simulink library "packLibrary"  (R2022b)
settings: Solver=VariableStepAuto  StartTime=0.0  StopTime=10.0  RelTol=1e-3
undefined symbols (not defined in the file or in its folder): battery_builder_rtmsupport, gcbh
libraries: packLibrary_lib x42
(part 4 of 4)

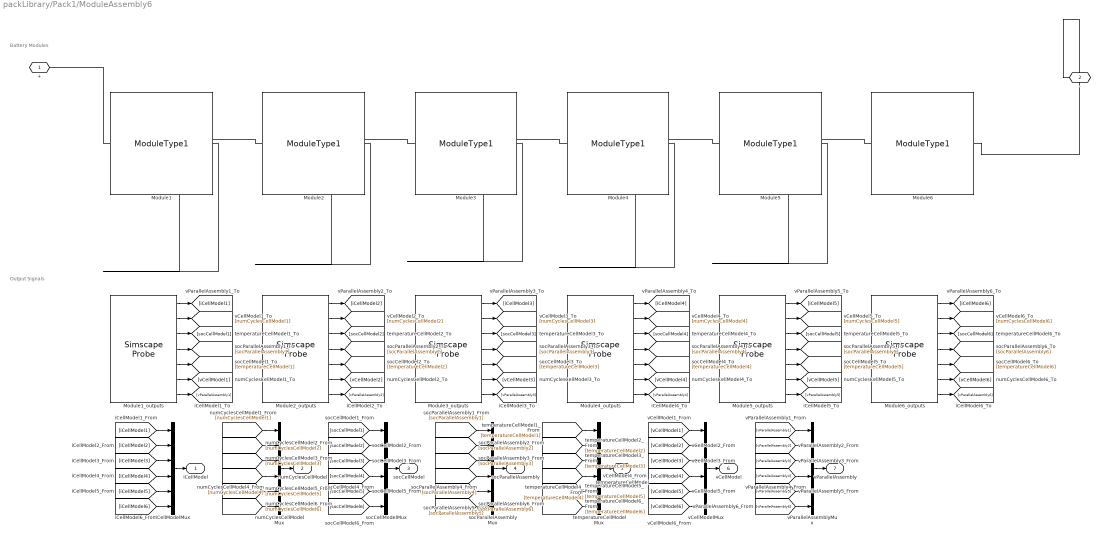
== system packLibrary/Pack1/ModuleAssembly6 ==
  note: Output Signals
  note: Battery Modules
  Module1 : packLibrary_lib/Modules/ModuleType1  SOC_vec=ModuleType1.SOC_vec  T_vec=ModuleType1.T_vec K  V0_mat=ModuleType1.V0_mat V  V_range=ModuleType1.V_range V  R0_mat=ModuleType1.R0_mat Ohm  AH=ModuleType1.AH A*hr  extrapolation_option=simscape.enum.extrapolation.nearest  thermal_mass=ModuleType1.thermal_mass J/K  P=4  S=3  iCellModel_specify=on  iCellModel_priority=None  iCellModel=ModuleAssembly6.Module1.iCellModel A  iCellModel_nominal_specify=off  iCellModel_nominal_unit=A  iCellModel_nominal_value=1  vCellModel_specify=on  vCellModel_priority=None  vCellModel=ModuleAssembly6.Module1.vCellModel V  vCellModel_nominal_specify=off  vCellModel_nominal_unit=V  vCellModel_nominal_value=1  socCellModel_specify=on  socCellModel_priority=High  socCellModel=ModuleAssembly6.Module1.socCellModel  socCellModel_nominal_specify=off  socCellModel_nominal_unit=1  socCellModel_nominal_value=1  numCyclesCellModel_specify=on  numCyclesCellModel_priority=High  numCyclesCellModel=ModuleAssembly6.Module1.numCyclesCellModel  numCyclesCellModel_nominal_specify=off  numCyclesCellModel_nominal_unit=1  numCyclesCellModel_nominal_value=1  temperatureCellModel_specify=on  temperatureCellModel_priority=High  temperatureCellModel=ModuleAssembly6.Module1.temperatureCellModel K  temperatureCellModel_nominal_specify=off  temperatureCellModel_nominal_unit=K  temperatureCellModel_nominal_value=1  vParallelAssembly_specify=on  vParallelAssembly_priority=None  vParallelAssembly=ModuleAssembly6.Module1.vParallelAssembly V  vParallelAssembly_nominal_specify=off  vParallelAssembly_nominal_unit=V  vParallelAssembly_nominal_value=1  socParallelAssembly_specify=on  socParallelAssembly_priority=None  socParallelAssembly=ModuleAssembly6.Module1.socParallelAssembly  socParallelAssembly_nominal_specify=off  socParallelAssembly_nominal_unit=1  socParallelAssembly_nominal_value=1
      settings: InternalSimscapePortConfiguration="{\"Bottom\":[{\"id\":\"n\",\"label\":\"-\",\"type\":\"foundation.electrical.electrical\"}],\"Left\":[],\"Right\":[],\"Top\":[{\"id\":\"p\",\"label\":\"+\",\"type\":\"foundation.electrical.electrical\"}]}"
  Module1_outputs : SimscapeProbe  BoundBlock=694  Variables={iCellModel, numCyclesCellModel, socCellModel, socParallelAssembly, temperatureCellModel, vCellModel, vParallelAssembly}
  Module2 : packLibrary_lib/Modules/ModuleType1  SOC_vec=ModuleType1.SOC_vec  T_vec=ModuleType1.T_vec K  V0_mat=ModuleType1.V0_mat V  V_range=ModuleType1.V_range V  R0_mat=ModuleType1.R0_mat Ohm  AH=ModuleType1.AH A*hr  extrapolation_option=simscape.enum.extrapolation.nearest  thermal_mass=ModuleType1.thermal_mass J/K  P=4  S=3  iCellModel_specify=on  iCellModel_priority=None  iCellModel=ModuleAssembly6.Module2.iCellModel A  iCellModel_nominal_specify=off  iCellModel_nominal_unit=A  iCellModel_nominal_value=1  vCellModel_specify=on  vCellModel_priority=None  vCellModel=ModuleAssembly6.Module2.vCellModel V  vCellModel_nominal_specify=off  vCellModel_nominal_unit=V  vCellModel_nominal_value=1  socCellModel_specify=on  socCellModel_priority=High  socCellModel=ModuleAssembly6.Module2.socCellModel  socCellModel_nominal_specify=off  socCellModel_nominal_unit=1  socCellModel_nominal_value=1  numCyclesCellModel_specify=on  numCyclesCellModel_priority=High  numCyclesCellModel=ModuleAssembly6.Module2.numCyclesCellModel  numCyclesCellModel_nominal_specify=off  numCyclesCellModel_nominal_unit=1  numCyclesCellModel_nominal_value=1  temperatureCellModel_specify=on  temperatureCellModel_priority=High  temperatureCellModel=ModuleAssembly6.Module2.temperatureCellModel K  temperatureCellModel_nominal_specify=off  temperatureCellModel_nominal_unit=K  temperatureCellModel_nominal_value=1  vParallelAssembly_specify=on  vParallelAssembly_priority=None  vParallelAssembly=ModuleAssembly6.Module2.vParallelAssembly V  vParallelAssembly_nominal_specify=off  vParallelAssembly_nominal_unit=V  vParallelAssembly_nominal_value=1  socParallelAssembly_specify=on  socParallelAssembly_priority=None  socParallelAssembly=ModuleAssembly6.Module2.socParallelAssembly  socParallelAssembly_nominal_specify=off  socParallelAssembly_nominal_unit=1  socParallelAssembly_nominal_value=1
      settings: InternalSimscapePortConfiguration="{\"Bottom\":[{\"id\":\"n\",\"label\":\"-\",\"type\":\"foundation.electrical.electrical\"}],\"Left\":[],\"Right\":[],\"Top\":[{\"id\":\"p\",\"label\":\"+\",\"type\":\"foundation.electrical.electrical\"}]}"
  Module2_outputs : SimscapeProbe  BoundBlock=696  Variables={iCellModel, numCyclesCellModel, socCellModel, socParallelAssembly, temperatureCellModel, vCellModel, vParallelAssembly}
  Module3 : packLibrary_lib/Modules/ModuleType1  SOC_vec=ModuleType1.SOC_vec  T_vec=ModuleType1.T_vec K  V0_mat=ModuleType1.V0_mat V  V_range=ModuleType1.V_range V  R0_mat=ModuleType1.R0_mat Ohm  AH=ModuleType1.AH A*hr  extrapolation_option=simscape.enum.extrapolation.nearest  thermal_mass=ModuleType1.thermal_mass J/K  P=4  S=3  iCellModel_specify=on  iCellModel_priority=None  iCellModel=ModuleAssembly6.Module3.iCellModel A  iCellModel_nominal_specify=off  iCellModel_nominal_unit=A  iCellModel_nominal_value=1  vCellModel_specify=on  vCellModel_priority=None  vCellModel=ModuleAssembly6.Module3.vCellModel V  vCellModel_nominal_specify=off  vCellModel_nominal_unit=V  vCellModel_nominal_value=1  socCellModel_specify=on  socCellModel_priority=High  socCellModel=ModuleAssembly6.Module3.socCellModel  socCellModel_nominal_specify=off  socCellModel_nominal_unit=1  socCellModel_nominal_value=1  numCyclesCellModel_specify=on  numCyclesCellModel_priority=High  numCyclesCellModel=ModuleAssembly6.Module3.numCyclesCellModel  numCyclesCellModel_nominal_specify=off  numCyclesCellModel_nominal_unit=1  numCyclesCellModel_nominal_value=1  temperatureCellModel_specify=on  temperatureCellModel_priority=High  temperatureCellModel=ModuleAssembly6.Module3.temperatureCellModel K  temperatureCellModel_nominal_specify=off  temperatureCellModel_nominal_unit=K  temperatureCellModel_nominal_value=1  vParallelAssembly_specify=on  vParallelAssembly_priority=None  vParallelAssembly=ModuleAssembly6.Module3.vParallelAssembly V  vParallelAssembly_nominal_specify=off  vParallelAssembly_nominal_unit=V  vParallelAssembly_nominal_value=1  socParallelAssembly_specify=on  socParallelAssembly_priority=None  socParallelAssembly=ModuleAssembly6.Module3.socParallelAssembly  socParallelAssembly_nominal_specify=off  socParallelAssembly_nominal_unit=1  socParallelAssembly_nominal_value=1
      settings: InternalSimscapePortConfiguration="{\"Bottom\":[{\"id\":\"n\",\"label\":\"-\",\"type\":\"foundation.electrical.electrical\"}],\"Left\":[],\"Right\":[],\"Top\":[{\"id\":\"p\",\"label\":\"+\",\"type\":\"foundation.electrical.electrical\"}]}"
  Module3_outputs : SimscapeProbe  BoundBlock=698  Variables={iCellModel, numCyclesCellModel, socCellModel, socParallelAssembly, temperatureCellModel, vCellModel, vParallelAssembly}
  Module4 : packLibrary_lib/Modules/ModuleType1  SOC_vec=ModuleType1.SOC_vec  T_vec=ModuleType1.T_vec K  V0_mat=ModuleType1.V0_mat V  V_range=ModuleType1.V_range V  R0_mat=ModuleType1.R0_mat Ohm  AH=ModuleType1.AH A*hr  extrapolation_option=simscape.enum.extrapolation.nearest  thermal_mass=ModuleType1.thermal_mass J/K  P=4  S=3  iCellModel_specify=on  iCellModel_priority=None  iCellModel=ModuleAssembly6.Module4.iCellModel A  iCellModel_nominal_specify=off  iCellModel_nominal_unit=A  iCellModel_nominal_value=1  vCellModel_specify=on  vCellModel_priority=None  vCellModel=ModuleAssembly6.Module4.vCellModel V  vCellModel_nominal_specify=off  vCellModel_nominal_unit=V  vCellModel_nominal_value=1  socCellModel_specify=on  socCellModel_priority=High  socCellModel=ModuleAssembly6.Module4.socCellModel  socCellModel_nominal_specify=off  socCellModel_nominal_unit=1  socCellModel_nominal_value=1  numCyclesCellModel_specify=on  numCyclesCellModel_priority=High  numCyclesCellModel=ModuleAssembly6.Module4.numCyclesCellModel  numCyclesCellModel_nominal_specify=off  numCyclesCellModel_nominal_unit=1  numCyclesCellModel_nominal_value=1  temperatureCellModel_specify=on  temperatureCellModel_priority=High  temperatureCellModel=ModuleAssembly6.Module4.temperatureCellModel K  temperatureCellModel_nominal_specify=off  temperatureCellModel_nominal_unit=K  temperatureCellModel_nominal_value=1  vParallelAssembly_specify=on  vParallelAssembly_priority=None  vParallelAssembly=ModuleAssembly6.Module4.vParallelAssembly V  vParallelAssembly_nominal_specify=off  vParallelAssembly_nominal_unit=V  vParallelAssembly_nominal_value=1  socParallelAssembly_specify=on  socParallelAssembly_priority=None  socParallelAssembly=ModuleAssembly6.Module4.socParallelAssembly  socParallelAssembly_nominal_specify=off  socParallelAssembly_nominal_unit=1  socParallelAssembly_nominal_value=1
      settings: InternalSimscapePortConfiguration="{\"Bottom\":[{\"id\":\"n\",\"label\":\"-\",\"type\":\"foundation.electrical.electrical\"}],\"Left\":[],\"Right\":[],\"Top\":[{\"id\":\"p\",\"label\":\"+\",\"type\":\"foundation.electrical.electrical\"}]}"
  Module4_outputs : SimscapeProbe  BoundBlock=700  Variables={iCellModel, numCyclesCellModel, socCellModel, socParallelAssembly, temperatureCellModel, vCellModel, vParallelAssembly}
  Module5 : packLibrary_lib/Modules/ModuleType1  SOC_vec=ModuleType1.SOC_vec  T_vec=ModuleType1.T_vec K  V0_mat=ModuleType1.V0_mat V  V_range=ModuleType1.V_range V  R0_mat=ModuleType1.R0_mat Ohm  AH=ModuleType1.AH A*hr  extrapolation_option=simscape.enum.extrapolation.nearest  thermal_mass=ModuleType1.thermal_mass J/K  P=4  S=3  iCellModel_specify=on  iCellModel_priority=None  iCellModel=ModuleAssembly6.Module5.iCellModel A  iCellModel_nominal_specify=off  iCellModel_nominal_unit=A  iCellModel_nominal_value=1  vCellModel_specify=on  vCellModel_priority=None  vCellModel=ModuleAssembly6.Module5.vCellModel V  vCellModel_nominal_specify=off  vCellModel_nominal_unit=V  vCellModel_nominal_value=1  socCellModel_specify=on  socCellModel_priority=High  socCellModel=ModuleAssembly6.Module5.socCellModel  socCellModel_nominal_specify=off  socCellModel_nominal_unit=1  socCellModel_nominal_value=1  numCyclesCellModel_specify=on  numCyclesCellModel_priority=High  numCyclesCellModel=ModuleAssembly6.Module5.numCyclesCellModel  numCyclesCellModel_nominal_specify=off  numCyclesCellModel_nominal_unit=1  numCyclesCellModel_nominal_value=1  temperatureCellModel_specify=on  temperatureCellModel_priority=High  temperatureCellModel=ModuleAssembly6.Module5.temperatureCellModel K  temperatureCellModel_nominal_specify=off  temperatureCellModel_nominal_unit=K  temperatureCellModel_nominal_value=1  vParallelAssembly_specify=on  vParallelAssembly_priority=None  vParallelAssembly=ModuleAssembly6.Module5.vParallelAssembly V  vParallelAssembly_nominal_specify=off  vParallelAssembly_nominal_unit=V  vParallelAssembly_nominal_value=1  socParallelAssembly_specify=on  socParallelAssembly_priority=None  socParallelAssembly=ModuleAssembly6.Module5.socParallelAssembly  socParallelAssembly_nominal_specify=off  socParallelAssembly_nominal_unit=1  socParallelAssembly_nominal_value=1
      settings: InternalSimscapePortConfiguration="{\"Bottom\":[{\"id\":\"n\",\"label\":\"-\",\"type\":\"foundation.electrical.electrical\"}],\"Left\":[],\"Right\":[],\"Top\":[{\"id\":\"p\",\"label\":\"+\",\"type\":\"foundation.electrical.electrical\"}]}"
  Module5_outputs : SimscapeProbe  BoundBlock=702  Variables={iCellModel, numCyclesCellModel, socCellModel, socParallelAssembly, temperatureCellModel, vCellModel, vParallelAssembly}
  Module6 : packLibrary_lib/Modules/ModuleType1  SOC_vec=ModuleType1.SOC_vec  T_vec=ModuleType1.T_vec K  V0_mat=ModuleType1.V0_mat V  V_range=ModuleType1.V_range V  R0_mat=ModuleType1.R0_mat Ohm  AH=ModuleType1.AH A*hr  extrapolation_option=simscape.enum.extrapolation.nearest  thermal_mass=ModuleType1.thermal_mass J/K  P=4  S=3  iCellModel_specify=on  iCellModel_priority=None  iCellModel=ModuleAssembly6.Module6.iCellModel A  iCellModel_nominal_specify=off  iCellModel_nominal_unit=A  iCellModel_nominal_value=1  vCellModel_specify=on  vCellModel_priority=None  vCellModel=ModuleAssembly6.Module6.vCellModel V  vCellModel_nominal_specify=off  vCellModel_nominal_unit=V  vCellModel_nominal_value=1  socCellModel_specify=on  socCellModel_priority=High  socCellModel=ModuleAssembly6.Module6.socCellModel  socCellModel_nominal_specify=off  socCellModel_nominal_unit=1  socCellModel_nominal_value=1  numCyclesCellModel_specify=on  numCyclesCellModel_priority=High  numCyclesCellModel=ModuleAssembly6.Module6.numCyclesCellModel  numCyclesCellModel_nominal_specify=off  numCyclesCellModel_nominal_unit=1  numCyclesCellModel_nominal_value=1  temperatureCellModel_specify=on  temperatureCellModel_priority=High  temperatureCellModel=ModuleAssembly6.Module6.temperatureCellModel K  temperatureCellModel_nominal_specify=off  temperatureCellModel_nominal_unit=K  temperatureCellModel_nominal_value=1  vParallelAssembly_specify=on  vParallelAssembly_priority=None  vParallelAssembly=ModuleAssembly6.Module6.vParallelAssembly V  vParallelAssembly_nominal_specify=off  vParallelAssembly_nominal_unit=V  vParallelAssembly_nominal_value=1  socParallelAssembly_specify=on  socParallelAssembly_priority=None  socParallelAssembly=ModuleAssembly6.Module6.socParallelAssembly  socParallelAssembly_nominal_specify=off  socParallelAssembly_nominal_unit=1  socParallelAssembly_nominal_value=1
      settings: InternalSimscapePortConfiguration="{\"Bottom\":[{\"id\":\"n\",\"label\":\"-\",\"type\":\"foundation.electrical.electrical\"}],\"Left\":[],\"Right\":[],\"Top\":[{\"id\":\"p\",\"label\":\"+\",\"type\":\"foundation.electrical.electrical\"}]}"
  Module6_outputs : SimscapeProbe  BoundBlock=704  Variables={iCellModel, numCyclesCellModel, socCellModel, socParallelAssembly, temperatureCellModel, vCellModel, vParallelAssembly}
  iCellModelMux : Mux  Inputs=6
  numCyclesCellModelMux : Mux  Inputs=6
  socCellModelMux : Mux  Inputs=6
  socParallelAssemblyMux : Mux  Inputs=6
  temperatureCellModelMux : Mux  Inputs=6
  vCellModelMux : Mux  Inputs=6
  vParallelAssemblyMux : Mux  Inputs=6
  + : PMIOPort  Side=Left
  - : PMIOPort  Port=2  Side=Right
  iCellModel : Outport
  numCyclesCellModel : Outport  Port=2
  socCellModel : Outport  Port=3
  socParallelAssembly : Outport  Port=4
  temperatureCellModel : Outport  Port=5
  vCellModel : Outport  Port=6
  vParallelAssembly : Outport  Port=7
  wires:
  [vParallelAssembly6] -> vParallelAssemblyMux/6
  Module6_outputs/1 -> [iCellModel6]
  [vCellModel6] -> vCellModelMux/6
  Module6_outputs/2 -> [numCyclesCellModel6]
  [temperatureCellModel6] -> temperatureCellModelMux/6
  Module6_outputs/3 -> [socCellModel6]
  [socParallelAssembly6] -> socParallelAssemblyMux/6
  Module6_outputs/4 -> [socParallelAssembly6]
  [socCellModel6] -> socCellModelMux/6
  Module6_outputs/5 -> [temperatureCellModel6]
  [numCyclesCellModel6] -> numCyclesCellModelMux/6
  Module6_outputs/6 -> [vCellModel6]
  [iCellModel6] -> iCellModelMux/6
  Module6_outputs/7 -> [vParallelAssembly6]
  [vParallelAssembly5] -> vParallelAssemblyMux/5
  Module5_outputs/1 -> [iCellModel5]
  [vCellModel5] -> vCellModelMux/5
  Module5_outputs/2 -> [numCyclesCellModel5]
  [temperatureCellModel5] -> temperatureCellModelMux/5
  Module5_outputs/3 -> [socCellModel5]
  [socParallelAssembly5] -> socParallelAssemblyMux/5
  Module5_outputs/4 -> [socParallelAssembly5]
  [socCellModel5] -> socCellModelMux/5
  Module5_outputs/5 -> [temperatureCellModel5]
  [numCyclesCellModel5] -> numCyclesCellModelMux/5
  Module5_outputs/6 -> [vCellModel5]
  [iCellModel5] -> iCellModelMux/5
  Module5_outputs/7 -> [vParallelAssembly5]
  [vParallelAssembly4] -> vParallelAssemblyMux/4
  Module4_outputs/1 -> [iCellModel4]
  [vCellModel4] -> vCellModelMux/4
  Module4_outputs/2 -> [numCyclesCellModel4]
  [temperatureCellModel4] -> temperatureCellModelMux/4
  Module4_outputs/3 -> [socCellModel4]
  [socParallelAssembly4] -> socParallelAssemblyMux/4
  Module4_outputs/4 -> [socParallelAssembly4]
  [socCellModel4] -> socCellModelMux/4
  Module4_outputs/5 -> [temperatureCellModel4]
  [numCyclesCellModel4] -> numCyclesCellModelMux/4
  Module4_outputs/6 -> [vCellModel4]
  [iCellModel4] -> iCellModelMux/4
  Module4_outputs/7 -> [vParallelAssembly4]
  [vParallelAssembly3] -> vParallelAssemblyMux/3
  Module3_outputs/1 -> [iCellModel3]
  [vCellModel3] -> vCellModelMux/3
  Module3_outputs/2 -> [numCyclesCellModel3]
  [temperatureCellModel3] -> temperatureCellModelMux/3
  Module3_outputs/3 -> [socCellModel3]
  [socParallelAssembly3] -> socParallelAssemblyMux/3
  Module3_outputs/4 -> [socParallelAssembly3]
  [socCellModel3] -> socCellModelMux/3
  Module3_outputs/5 -> [temperatureCellModel3]
  [numCyclesCellModel3] -> numCyclesCellModelMux/3
  Module3_outputs/6 -> [vCellModel3]
  [iCellModel3] -> iCellModelMux/3
  Module3_outputs/7 -> [vParallelAssembly3]
  [vParallelAssembly2] -> vParallelAssemblyMux/2
  Module2_outputs/1 -> [iCellModel2]
  [vCellModel2] -> vCellModelMux/2
  Module2_outputs/2 -> [numCyclesCellModel2]
  [temperatureCellModel2] -> temperatureCellModelMux/2
  Module2_outputs/3 -> [socCellModel2]
  [socParallelAssembly2] -> socParallelAssemblyMux/2
  Module2_outputs/4 -> [socParallelAssembly2]
  [socCellModel2] -> socCellModelMux/2
  Module2_outputs/5 -> [temperatureCellModel2]
  [numCyclesCellModel2] -> numCyclesCellModelMux/2
  Module2_outputs/6 -> [vCellModel2]
  [iCellModel2] -> iCellModelMux/2
  Module2_outputs/7 -> [vParallelAssembly2]
  [vParallelAssembly1] -> vParallelAssemblyMux/1
  vParallelAssemblyMux/1 -> vParallelAssembly/1
  Module1_outputs/1 -> [iCellModel1]
  [vCellModel1] -> vCellModelMux/1
  vCellModelMux/1 -> vCellModel/1
  Module1_outputs/2 -> [numCyclesCellModel1]
  [temperatureCellModel1] -> temperatureCellModelMux/1
  temperatureCellModelMux/1 -> temperatureCellModel/1
  Module1_outputs/3 -> [socCellModel1]
  [socParallelAssembly1] -> socParallelAssemblyMux/1
  socParallelAssemblyMux/1 -> socParallelAssembly/1
  Module1_outputs/4 -> [socParallelAssembly1]
  [socCellModel1] -> socCellModelMux/1
  socCellModelMux/1 -> socCellModel/1
  Module1_outputs/5 -> [temperatureCellModel1]
  [numCyclesCellModel1] -> numCyclesCellModelMux/1
  numCyclesCellModelMux/1 -> numCyclesCellModel/1
  Module1_outputs/6 -> [vCellModel1]
  [iCellModel1] -> iCellModelMux/1
  iCellModelMux/1 -> iCellModel/1
  Module1_outputs/7 -> [vParallelAssembly1]
  connections:
  Module6/RConn1 -- -/RConn1
  Module1/LConn1 -- +/RConn1
  Module6/LConn1 -- Module5/RConn1
  Module5/LConn1 -- Module4/RConn1
  Module4/LConn1 -- Module3/RConn1
  Module3/LConn1 -- Module2/RConn1
  Module2/LConn1 -- Module1/RConn1
